simulink model "lego2"  (R2016a)
settings: Solver=VariableStepAuto  SolverMode=SingleTasking  StartTime=0.0  StopTime=inf  RelTol=1e-3
libraries: simulink x10, legonxtlib x6
settings Model: SimulationMode=external  ExtModeTrigDuration=2  Creator=Luka  LastModifiedBy=Lovro
settings OptimizationCC: OptimizeModelRefInitCode=on  LifeSpan=Inf
settings HardwareCC: ProdBitPerPointer=32  ProdLargestAtomicInteger=Long  ProdWordSize=32  ProdHWDeviceType=ARM Compatible->ARM 7
settings RTWCC: SystemTargetFile=realtime.tlc  GenerateMakefile=off  TemplateMakefile=realtime.tmf  Description=Run on Target Hardware  RTWVerbose=off  IncludeHyperlinkInReport=on
settings CodeAppCC: ForceParamTrailComments=on  OperatorAnnotations=on  SimulinkDataObjDesc=on  SFDataObjDesc=on  MATLABFcnDesc=on  InsertBlockDesc=on  MATLABSourceComments=on
settings STFCustomTargetCC: TargetLibSuffix=.a  GenerateSampleERTMain=on  ERTCustomFileBanners=on  SupportNonInlinedSFcns=off  SupportVariableSizeSignals=on  MATLABClassNameForMDSCustomization=Simulink.SoftwareTarget.ERTCustomization  GRTInterface=off  SystemTargetFile=realtime.tlc
settings ERTTargetCC: GenerateSampleERTMain=on  ParMdlRefBuildCompliant=off  CompOptLevelCompliant=off  ConcurrentExecutionCompliant=off  CombineOutputUpdateFcns=off  ERTFirstTimeCompliant=off  SupportContinuousTime=on  SupportVariableSizeSignals=on  ModelStepFunctionPrototypeControlCompliant=off  CPPClassGenCompliant=off  UseToolchainInfoCompliant=off  ExtMode=on  ExtModeTransport=3  ExtModeMexFile=ext_serial_win32_comm_rtt  ExtModeMexArgs=0 3 9600  ERTSrcFileBannerTemplate=realtime_code_template.cgt  ERTHdrFileBannerTemplate=realtime_code_template.cgt  ERTDataSrcFileTemplate=realtime_code_template.cgt  ERTDataHdrFileTemplate=realtime_code_template.cgt  ERTCustomFileTemplate=realtime_file_process.tlc

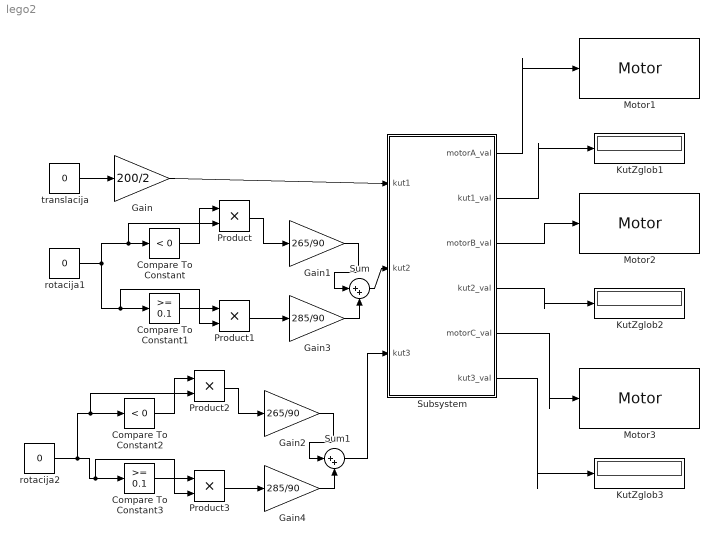
== system lego2 ==
  Compare To Constant : simulink/Logic and Bit Operations/Compare To Constant  relop=<  const=0  OutDataTypeStr=boolean
  Compare To Constant1 : simulink/Logic and Bit Operations/Compare To Constant  relop=>=  const=0.1  OutDataTypeStr=boolean
  Compare To Constant2 : simulink/Logic and Bit Operations/Compare To Constant  relop=<  const=0  OutDataTypeStr=boolean
  Compare To Constant3 : simulink/Logic and Bit Operations/Compare To Constant  relop=>=  const=0.1  OutDataTypeStr=boolean
  Gain : Gain  Gain=200/2
  Gain1 : Gain  Gain=265/90
  Gain2 : Gain  Gain=265/90
  Gain3 : Gain  Gain=285/90
  Gain4 : Gain  Gain=285/90
  KutZglob1 : Display
  KutZglob2 : Display
  KutZglob3 : Display
  Motor1 : legonxtlib/Motor  sportNumber=A  sstopAction=Brake  blockPlatform=LegoMindstormsNXT
  Motor2 : legonxtlib/Motor  sportNumber=B  sstopAction=Brake  blockPlatform=LegoMindstormsNXT
  Motor3 : legonxtlib/Motor  sportNumber=C  sstopAction=Brake  blockPlatform=LegoMindstormsNXT
  Product{,1..3} (4 alike) : Product
  Subsystem : Subsystem
  Sum : Sum  Inputs=|++
  Sum1 : Sum  Inputs=|++
  rotacija1 : Constant  Value=0
  rotacija2 : Constant  Value=0
  translacija : Constant  Value=0
  wires:
  translacija/1 -> Gain/1
  Subsystem/1(motorA_val) -> Motor1/1
  Subsystem/2(kut1_val) -> KutZglob1/1
  Subsystem/3(motorB_val) -> Motor2/1
  Subsystem/4(kut2_val) -> KutZglob2/1
  Subsystem/5(motorC_val) -> Motor3/1
  Subsystem/6(kut3_val) -> KutZglob3/1
  Gain/1 -> Subsystem/1(kut1)
  rotacija1/1 -> Product/2, Compare To Constant/1, Product1/2, Compare To Constant1/1
  Compare To Constant/1 -> Product/1
  Product/1 -> Gain1/1
  Compare To Constant1/1 -> Product1/1
  Gain3/1 -> Sum/2
  Gain1/1 -> Sum/1
  Sum/1 -> Subsystem/2(kut2)
  Product1/1 -> Gain3/1
  Compare To Constant2/1 -> Product2/1
  Product2/1 -> Gain2/1
  Compare To Constant3/1 -> Product3/1
  Gain4/1 -> Sum1/2
  Product3/1 -> Gain4/1
  rotacija2/1 -> Product2/2, Compare To Constant2/1, Product3/2, Compare To Constant3/1
  Sum1/1 -> Subsystem/3(kut3)
  Gain2/1 -> Sum1/1

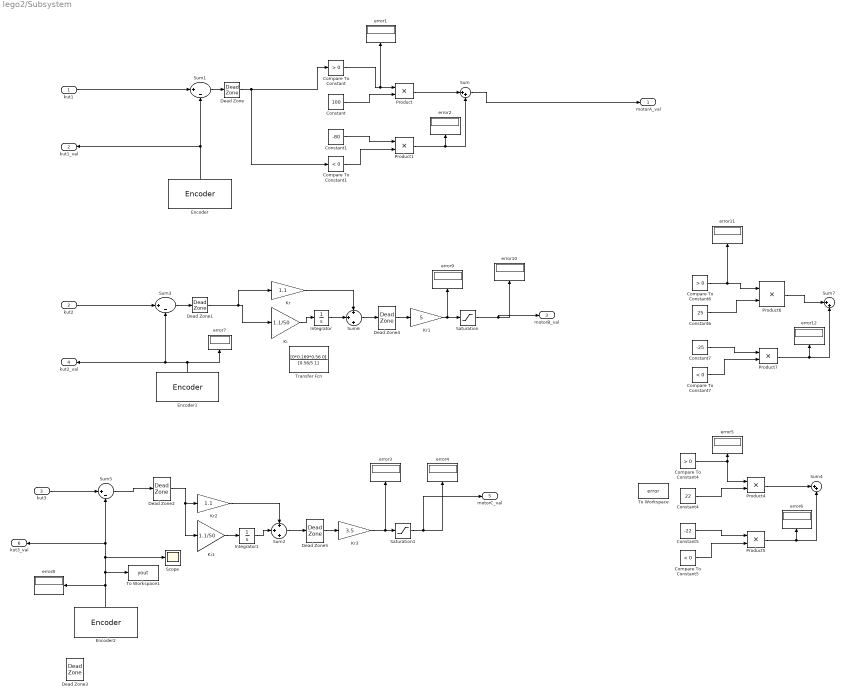
== system lego2/Subsystem ==
  kut1 : Inport
  kut2 : Inport  Port=2
  kut3 : Inport  Port=3
  Compare To Constant : simulink/Logic and Bit Operations/Compare To Constant  relop=>  const=0  OutDataTypeStr=uint8
  Compare To Constant1 : simulink/Logic and Bit Operations/Compare To Constant  relop=<  const=0  OutDataTypeStr=uint8
  Compare To Constant4 : simulink/Logic and Bit Operations/Compare To Constant  relop=>  const=0  OutDataTypeStr=uint8
  Compare To Constant5 : simulink/Logic and Bit Operations/Compare To Constant  relop=<  const=0  OutDataTypeStr=uint8
  Compare To Constant6 : simulink/Logic and Bit Operations/Compare To Constant  relop=>  const=0  OutDataTypeStr=uint8
  Compare To Constant7 : simulink/Logic and Bit Operations/Compare To Constant  relop=<  const=0  OutDataTypeStr=uint8
  Constant : Constant  Value=100
  Constant1 : Constant  Value=-80
  Constant4 : Constant  Value=22
  Constant5 : Constant  Value=-22
  Constant6 : Constant  Value=25
  Constant7 : Constant  Value=-25
  Dead Zone : DeadZone  LowerValue=-50  UpperValue=50  LinearizeAsGain=off  SaturateOnIntegerOverflow=on
  Dead Zone1 : DeadZone  LowerValue=0  UpperValue=0  LinearizeAsGain=off  SaturateOnIntegerOverflow=on
  Dead Zone2 : DeadZone  LowerValue=0  UpperValue=0  LinearizeAsGain=off  SaturateOnIntegerOverflow=on
  Dead Zone3 : DeadZone  LowerValue=-4  UpperValue=4  LinearizeAsGain=off  SaturateOnIntegerOverflow=on
  Dead Zone4 : DeadZone  LinearizeAsGain=off  SaturateOnIntegerOverflow=on
  Dead Zone5 : DeadZone  LinearizeAsGain=off  SaturateOnIntegerOverflow=on
  Encoder : legonxtlib/Encoder  portNumber=A  opMode=No reset  sampleTime=0.1  blockPlatform=LegoMindstormsNXT
  Encoder1 : legonxtlib/Encoder  portNumber=B  opMode=No reset  sampleTime=0.1  blockPlatform=LegoMindstormsNXT
  Encoder2 : legonxtlib/Encoder  portNumber=C  opMode=No reset  sampleTime=0.1  blockPlatform=LegoMindstormsNXT
  Integrator : Integrator
  Integrator1 : Integrator
  Ki : Gain  Gain=1.1/50
  Ki1 : Gain  Gain=1.1/50
  Kr : Gain  Gain=1.1
  Kr1 : Gain  Gain=5
  Kr2 : Gain  Gain=1.1
  Kr3 : Gain  Gain=3.5
  Product{,1,4..7} (6 alike) : Product
  Saturation : Saturate  UpperLimit=25  LowerLimit=-25
  Saturation1 : Saturate  UpperLimit=35  LowerLimit=-35
  Scope : Scope
  Sum : Sum  Inputs=|++
  Sum1 : Sum  Inputs=|+-
  Sum2 : Sum  Inputs=+|+|+
  Sum3 : Sum  Inputs=|+-
  Sum4 : Sum  Inputs=|++
  Sum5 : Sum  Inputs=|+-
  Sum6 : Sum  Inputs=+|+|+
  Sum7 : Sum  Inputs=|++
  To Workspace : ToWorkspace  VariableName=error  SaveFormat=Structure With Time  SampleTime=-1
  To Workspace1 : ToWorkspace  VariableName=yout  SampleTime=-1
  Transfer Fcn : TransferFcn  Numerator=[0*0.169*0.56 0]  Denominator=[0.56/5 1]
  error{1..12} (12 alike) : Display
  motorA_val : Outport
  kut1_val : Outport  Port=2
  motorB_val : Outport  Port=3
  kut2_val : Outport  Port=4
  motorC_val : Outport  Port=5
  kut3_val : Outport  Port=6
  wires:
  kut2/1 -> Sum3/1
  Encoder1/1 -> error7/1, kut2_val/1, Sum3/2
  Sum3/1 -> Dead Zone1/1
  Compare To Constant4/1 -> Product4/1, error5/1
  Constant4/1 -> Product4/2
  Product4/1 -> Sum4/1
  kut3/1 -> Sum5/1
  Constant5/1 -> Product5/1
  Product5/1 -> error6/1, Sum4/2
  Compare To Constant5/1 -> Product5/2
  Constant1/1 -> Product1/1
  Encoder/1 -> kut1_val/1, Sum1/2
  kut1/1 -> Sum1/1
  Compare To Constant/1 -> error1/1, Product/1
  Sum/1 -> motorA_val/1
  Constant/1 -> Product/2
  Dead Zone/1 -> Compare To Constant1/1, Compare To Constant/1
  Sum1/1 -> Dead Zone/1
  Compare To Constant1/1 -> Product1/2
  Product/1 -> Sum/1
  Product1/1 -> error2/1, Sum/2
  Kr/1 -> Sum6/1
  Integrator/1 -> Sum6/2
  Encoder2/1 -> kut3_val/1, Sum5/2, Scope/1, To Workspace1/1, error8/1
  Sum5/1 -> Dead Zone2/1
  Sum6/1 -> Dead Zone4/1
  Saturation/1 -> motorB_val/1, error10/1
  Dead Zone4/1 -> Kr1/1
  Kr1/1 -> Saturation/1, error9/1
  Product6/1 -> Sum7/1
  Product7/1 -> Sum7/2, error12/1
  Compare To Constant7/1 -> Product7/2
  Constant7/1 -> Product7/1
  Constant6/1 -> Product6/2
  Compare To Constant6/1 -> error11/1, Product6/1
  Kr2/1 -> Sum2/1
  Integrator1/1 -> Sum2/2
  Ki1/1 -> Integrator1/1
  Sum2/1 -> Dead Zone5/1
  Dead Zone5/1 -> Kr3/1
  Kr3/1 -> error3/1, Saturation1/1
  Saturation1/1 -> motorC_val/1, error4/1
  Dead Zone2/1 -> Ki1/1, Kr2/1
  Ki/1 -> Integrator/1
  Dead Zone1/1 -> Kr/1, Ki/1
